simulink model "can_git"  (R2022a)
settings: Solver=FixedStepAuto  StartTime=0.0  StopTime=inf  FixedStep=0.005  RelTol=1e-3
undefined symbols (not defined in the file): Down, Pull
libraries: speedgoatlib_IO691 x3, canmsglib x2
settings Model: Creator=luanb  LastModifiedBy=luanb
settings SolverCC: ConcurrentTasks=on  PositivePriorityOrder=on  AutoInsertRateTranBlk=on  InsertRTBMode=Never (minimum delay)
settings OptimizationCC: BlockReduction=off  OptimizeBlockIOStorage=off  InitFltsAndDblsToZero=on
settings DebuggingCC: TasksWithSamePriorityMsg=none
settings HardwareCC: ProdBitPerLong=64  ProdLongLongMode=on  ProdHWDeviceType=Intel->x86-64 (Linux 64)  TargetLongLongMode=on
settings RTWCC: Description=Simulink Real-Time  SystemTargetFile=slrealtime.tlc  TemplateMakefile=slrealtime_default_tmf  Toolchain=Simulink Real-Time Toolchain  BuildConfiguration=Faster Runs  CodeExecutionProfiling=on  TargetLang=C++
settings SimulinkRealTimeTargetCC: SLRTForcePollingMode=on  UseGCCFastMath=on

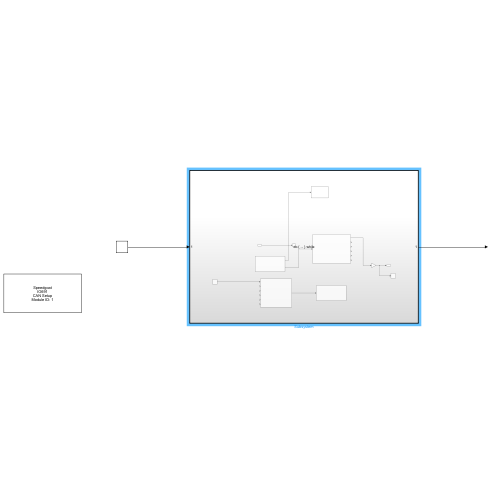
[thumbnail: Simulink's stored preview of the top-level diagram]
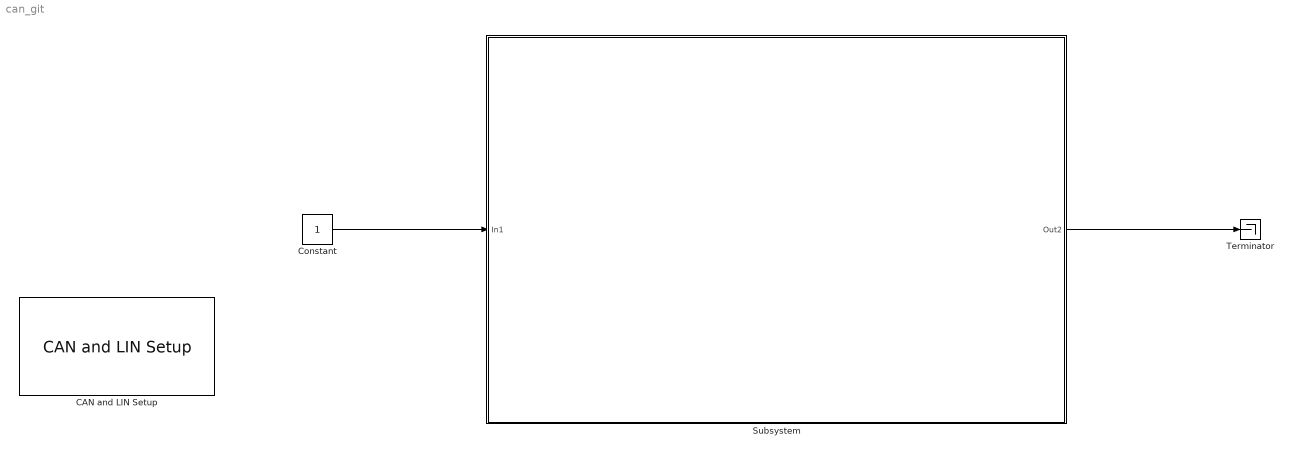
== system can_git ==
  "CAN and LIN Setup " : speedgoatlib_IO691/CAN and LIN Setup   moduleInitValues="[691    1    1   -1   -1]"  id=1  moduleType=IO691  pciSlot=-1  canChn1=CAN (HS)  canChn2=CAN (HS)  canChn3=Disabled  canChn4=Disabled  linChn1=Disabled  linChn2=Disabled  canInitStructArray=[]  canTermStructArray=[]  gpioChnx=Disabled  canChn1InitValues="[2   0   4   1  16   3  19   2   2   5   2   0]"  arbBdrChn1=1.0 MBaud  clockDividerChn1=Enable  arbManBdrChn1=[4,1,16,3]  fdBdrChn1=5.0 MBaud  fdManBdrChn1=[2,2,5,2]  termResistor1=off  canChn2InitValues="[2   0   4   1  16   3  19   2   2   5   2   0]"  arbBdrChn2=1.0 MBaud  clockDividerChn2=Enable  arbManBdrChn2=[4,1,16,3]  fdBdrChn2=5.0 MBaud  fdManBdrChn2=[2,2,5,2]  termResistor2=off  canChn3InitValues="[1   0   2   8  31   8  19   2   2   5   2   0]"  arbBdrChn3=1.0 MBaud  clockDividerChn3=Enable  arbManBdrChn3=[2,8,31,8]  fdBdrChn3=5.0 MBaud  fdManBdrChn3=[2,2,5,2]  termResistor3=off  canChn4InitValues="[1   0   2   8  31   8  19   2   2   5   2   0]"  arbBdrChn4=1.0 MBaud  clockDividerChn4=Enable  arbManBdrChn4=[2,8,31,8]  fdBdrChn4=5.0 MBaud  fdManBdrChn4=[2,2,5,2]  termResistor4=off  linChn1InitValues="[0  9600]"  linBtrChn1=9600  linChn2InitValues="[0  9600]"  linBtrChn2=9600  doInitTermStruct="[0  5  0  0  0]"  parDoChannels=[1 2]  parDoVoltage=5  parDoInitValues=0  parDoReset=1  parNumOfDoS=0  parDiChannels=[3 4]  parDiVoltage=5  parDiPull=Pull-Down
      settings: SourceProductName=Simulink Real-Time: Speedgoat I/O Blockset
  Constant : Constant  SampleTime=0.005
  Subsystem : Subsystem
  Terminator : Terminator
  wires:
  Constant/1 -> Subsystem/1(In1)
  Subsystem/1(Out2) -> Terminator/1

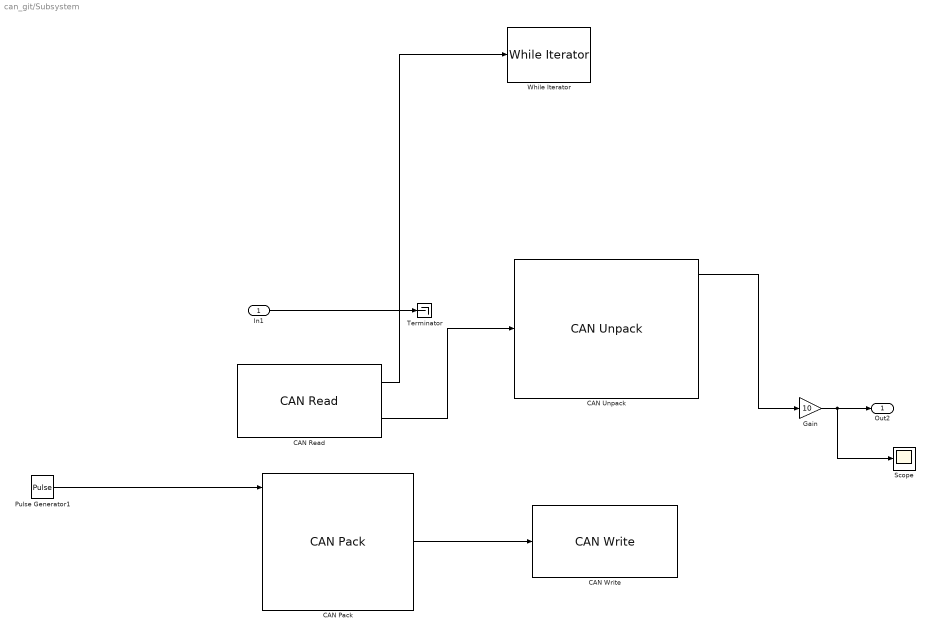
== system can_git/Subsystem ==
  In1 : Inport
  CAN Pack : canmsglib/CAN Pack  CANdbFile=C:\Users\luanb\Downloads\CAN_DB_dufour_v1 (1).dbc  MsgList=temp_LV_cell  MsgName=temp_LV_cell  MsgIDType=Standard (11-bit identifier)  MsgIdentifier=903  MsgLength=6  Remote=off  ApplyMinMax=off  BusOutput=off  SignalInfo={'temp_LV_cell_1','0','8','BE','unsigned','Standard','0','1','0','2.3','97.925';'temp_LV_cell_2','8','8','BE','unsigned','Standard','0','1','0','2.3','97.925';'temp_LV_cell_3','16','8','BE','unsigned','Standard','0','1','0','2.3','97.925';'temp_LV_cell_4','24','8','BE','unsigned','Standard','0','1','0','2.3','97.925';'temp_LV_cell_5','32','8','BE','unsigned','Standard','0','1','0','2.3','97.925';'temp_LV_cell_6','40','8','BE','unsigned','Standard','0','1','0','2.3','97.925'}
      settings: SourceProductBaseCode=XP,ME,VN  DataFormat=CANdb specified signals
  "CAN Read " : speedgoatlib_IO691/CAN Read   moduleType=IO691  id=1  channel=1  canType=CAN (HS)  messageType=CAN (HS)  useBusOut=off  HasMulRead=Single Read from Buffer (FIFO)  MsgIDlist=[1,2,3]  isEFF=on  LabelInHex=on  enableInput=off  initValues=[691 1 -1 0 1 1 0 0 1 1 3 1 2 3]  ts=-1
      settings: SourceProductName=Simulink Real-Time: Speedgoat I/O Blockset
  CAN Unpack : canmsglib/CAN Unpack  CANdbFile=C:\Users\luanb\Downloads\CAN_DB_dufour_v1.dbc  MsgList=temp_LV_cell  MsgName=temp_LV_cell  MsgIDType=Standard (11-bit identifier)  MsgIdentifier=903  MsgLength=6  SignalInfo={'temp_LV_cell_1','0','8','BE','unsigned','Standard','0','1','0','2.3','97.925';'temp_LV_cell_2','8','8','BE','unsigned','Standard','0','1','0','2.3','97.925';'temp_LV_cell_3','16','8','BE','unsigned','Standard','0','1','0','2.3','97.925';'temp_LV_cell_4','24','8','BE','unsigned','Standard','0','1','0','2.3','97.925';'temp_LV_cell_5','32','8','BE','unsigned','Standard','0','1','0','2.3','97.925';'temp_LV_cell_6','40','8','BE','unsigned','Standard','0','1','0','2.3','97.925'}  IDPort=off  TimestampPort=off  ErrorPort=off  RemotePort=off  LengthPort=off  StatusPort=off  ApplyMinMax=off
      settings: SourceProductBaseCode=XP,ME,VN  DataFormat=CANdb specified signals
  "CAN Write " : speedgoatlib_IO691/CAN Write   moduleType=IO691  id=1  channel=2  canType=CAN (HS)  messageType=CAN (HS)  useBusIn=off  numOfMsg=1  enableInput=off  enableStatusPort=off  ts=-1  initValues=[691 1 -1 1 1 1 0 1 0 0]
      settings: SourceProductName=Simulink Real-Time: Speedgoat I/O Blockset
  Gain : Gain  Gain=10
  Pulse Generator1 : DiscretePulseGenerator  Period=1000  PulseWidth=500  SampleTime=-1
  Scope : Scope
  Terminator : Terminator
  While Iterator : WhileIterator  MaxIters=-1  WhileBlockType=do-while
  Out2 : Outport
  wires:
  In1/1 -> Terminator/1
  CAN Unpack/1 -> Gain/1
  Gain/1 -> Scope/1, Out2/1
  Pulse Generator1/1 -> CAN Pack/1
  "CAN Read "/1 -> While Iterator/1
  "CAN Read "/2 -> CAN Unpack/1
  CAN Pack/1 -> "CAN Write "/1
